simulink subsystem "VehicleSimulationRef1"  (R2020b)
settings: Solver=VariableStepAuto  StartTime=0.0  StopTime=10.0  RelTol=1e-3
libraries: simulink x1
settings Model: Creator=tbritton  LastModifiedBy=azmol

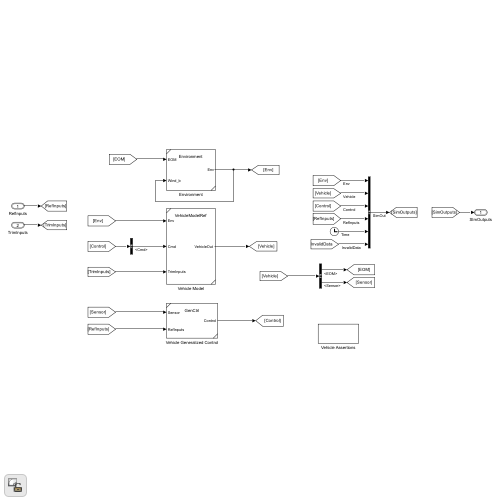
[thumbnail: Simulink's stored preview of the top-level diagram]
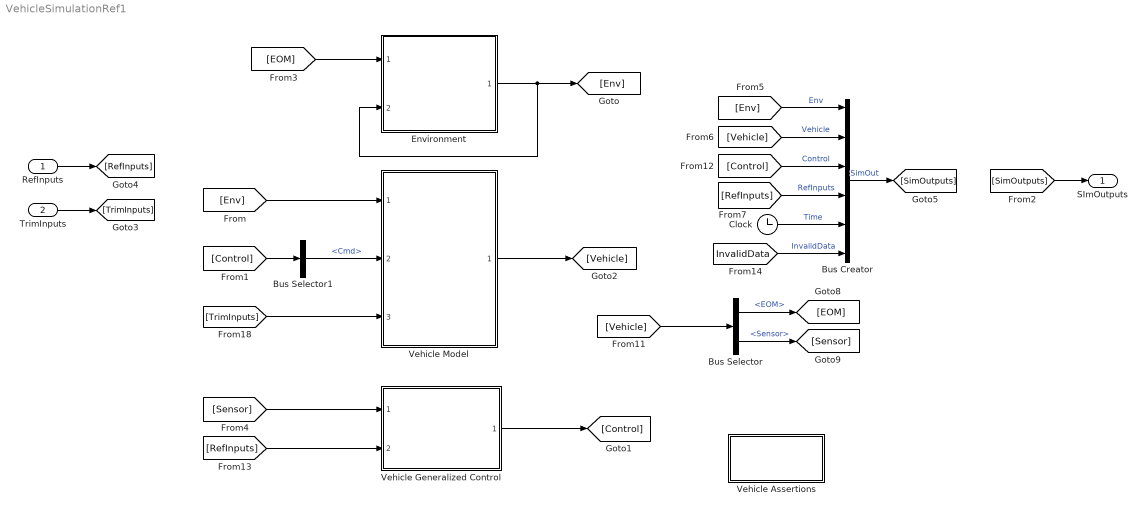
== system VehicleSimulationRef1 ==
  RefInputs : Inport  OutDataTypeStr=Bus: BUS_REF_INPUT
  TrimInputs : Inport  Port=2  OutDataTypeStr=Bus: BUS_TRIM_INPUT
  Bus Creator : BusCreator  Inputs=6  OutDataTypeStr=Bus: BUS_SIM_OUT  NonVirtualBus=on
  Bus Selector : BusSelector  OutputSignals=EOM,Sensor
  Bus Selector1 : BusSelector  OutputSignals=Cmd
  Clock : Clock
  Environment : Subsystem  ReferencedSubsystem=Environment
  Vehicle Assertions : Subsystem
  Vehicle Generalized Control : Subsystem  ReferencedSubsystem=GenCtrl
  Vehicle Model : Subsystem  ReferencedSubsystem=VehicleModelRef
  SImOutputs : Outport  OutDataTypeStr=Bus: BUS_SIM_OUT
  wires:
  [Sensor] -> Vehicle Generalized Control/1
  [Env] -> Bus Creator/1  "Env"
  [RefInputs] -> Bus Creator/4  "RefInputs"
  Environment/1 -> [Env], Environment/2
  Vehicle Generalized Control/1 -> [Control]
  [Vehicle] -> Bus Creator/2  "Vehicle"
  [Control] -> Bus Creator/3  "Control"
  Bus Selector/1 -> [EOM]  "<EOM>"
  [Vehicle] -> Bus Selector/1
  [EOM] -> Environment/1
  Bus Selector/2 -> [Sensor]  "<Sensor>"
  [Control] -> Bus Selector1/1
  [RefInputs] -> Vehicle Generalized Control/2
  Clock/1 -> Bus Creator/5  "Time"
  TrimInputs/1 -> [TrimInputs]
  RefInputs/1 -> [RefInputs]
  [SimOutputs] -> SImOutputs/1
  Bus Creator/1 -> [SimOutputs]  "SimOut"
  [InvalidData] -> Bus Creator/6  "InvalidData"
  [Env] -> Vehicle Model/1
  Bus Selector1/1 -> Vehicle Model/2  "<Cmd>"
  [TrimInputs] -> Vehicle Model/3
  Vehicle Model/1 -> [Vehicle]

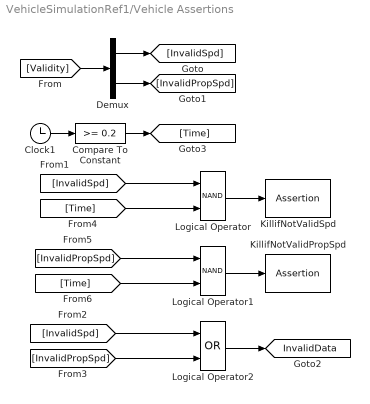
== system VehicleSimulationRef1/Vehicle Assertions ==
  Clock1 : Clock
  Compare To Constant : simulink/Logic and Bit Operations/Compare To Constant  relop=>=  const=0.2  OutDataTypeStr=boolean  ZeroCross=off
  Demux : Demux  Outputs=2
  KillifNotValidPropSpd : Assertion  AssertionFailFcn=warndlg('Model invalid prop speeds','Warning!')
  KillifNotValidSpd : Assertion  AssertionFailFcn=warndlg('Model invalid speed','Warning!')
  Logical Operator : Logic  Operator=NAND  AllPortsSameDT=off  OutDataTypeStr=boolean
  Logical Operator1 : Logic  Operator=NAND  AllPortsSameDT=off  OutDataTypeStr=boolean
  Logical Operator2 : Logic  Operator=OR  AllPortsSameDT=off  OutDataTypeStr=boolean
  tag scope: InvalidData=global
  wires:
  [InvalidPropSpd] -> Logical Operator2/2
  [InvalidSpd] -> Logical Operator2/1
  Logical Operator2/1 -> [InvalidData]
  Logical Operator/1 -> KillifNotValidSpd/1
  [InvalidPropSpd] -> Logical Operator1/1
  Logical Operator1/1 -> KillifNotValidPropSpd/1
  [Time] -> Logical Operator1/2
  [Time] -> Logical Operator/2
  Compare To Constant/1 -> [Time]
  Demux/2 -> [InvalidPropSpd]
  Demux/1 -> [InvalidSpd]
  [Validity] -> Demux/1
  [InvalidSpd] -> Logical Operator/1
  Clock1/1 -> Compare To Constant/1
